simulink model "estimate_gamma_fitting_param"  (R2022a)
settings: Solver=VariableStepAuto  StartTime=0.0  StopTime=tmax  RelTol=1e-3
values from neighbouring files (symbols this model uses):
  c2 = 5    [modelling_parameters.m]
  c2c = c2    (= 5)    [modelling_parameters.m]
  Cr = 2.5    [modelling_parameters.m]
  Eo = 8.41    [modelling_parameters.m]
  K1 = (Voc_min_mes-Eo+K2/soc_min)/-log(100-soc_min)    [modelling_parameters.m]
  K2 = (Voc_max_mes-Eo)*-soc_max    (= 0.99)    [modelling_parameters.m]
  K3 = 1*(-R0+R_soc_min)*soc_min    (= 0.416)    [modelling_parameters.m]
  K3c = 0.02*(-Rc+R_soc_minc)*soc_min    (= 0.00513333333333)    [modelling_parameters.m]
  K4 = 1*(-R0+R_soc_max)*(100-soc_max)    (= -1.45716771982e-16)    [modelling_parameters.m]
  K4c = 2*(-Rc+R_soc_maxc)*(100-soc_max)    (= 0.0733333333333)    [modelling_parameters.m]
  R0 = 0.04    [modelling_parameters.m]
  Rc = 0.03    [modelling_parameters.m]
  Ts = 0.2    [modelling_parameters.m]
settings Model: Creator=spinolam  LastModifiedBy=spinolam

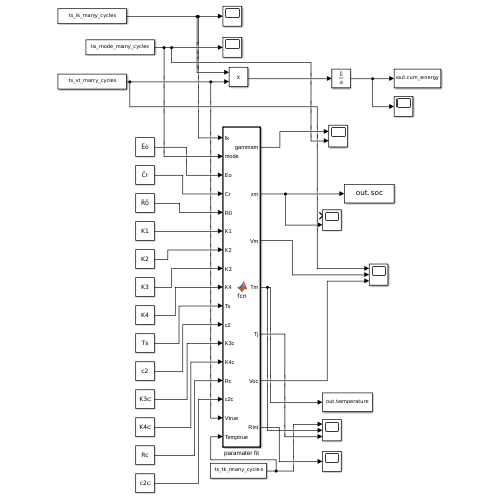
[thumbnail: Simulink's stored preview of the top-level diagram]
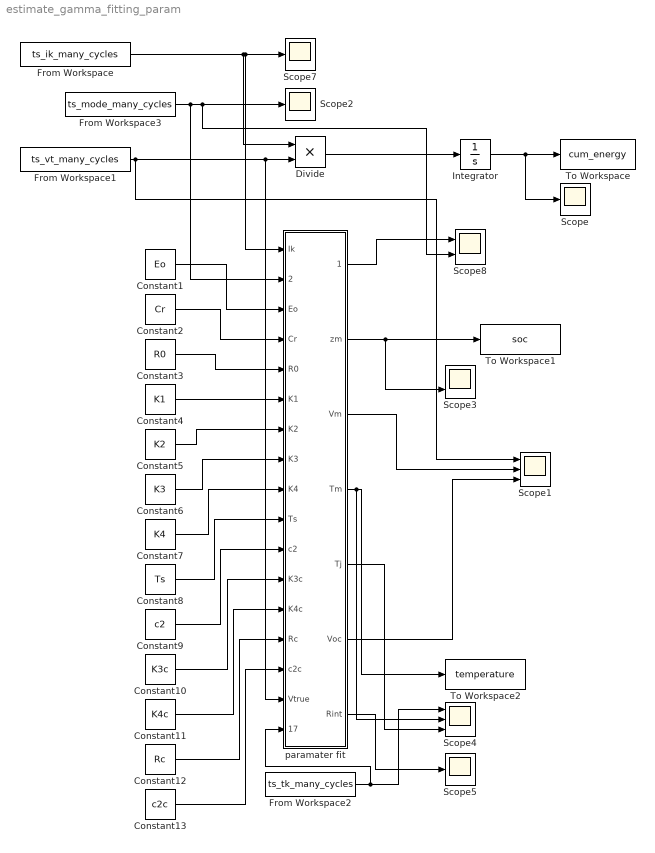
== system estimate_gamma_fitting_param ==
  Constant1 : Constant  Value=Eo
  Constant10 : Constant  Value=K3c
  Constant11 : Constant  Value=K4c
  Constant12 : Constant  Value=Rc
  Constant13 : Constant  Value=c2c
  Constant2 : Constant  Value=Cr
  Constant3 : Constant  Value=R0
  Constant4 : Constant  Value=K1
  Constant5 : Constant  Value=K2
  Constant6 : Constant  Value=K3
  Constant7 : Constant  Value=K4
  Constant8 : Constant  Value=Ts
  Constant9 : Constant  Value=c2
  Divide : Product  Inputs=**
  From Workspace : FromWorkspace  VariableName=ts_ik_many_cycles  SampleTime=Ts
  From Workspace1 : FromWorkspace  VariableName=ts_vt_many_cycles  SampleTime=Ts
  From Workspace2 : FromWorkspace  VariableName=ts_tk_many_cycles  SampleTime=1
  From Workspace3 : FromWorkspace  VariableName=ts_mode_many_cycles  SampleTime=Ts
  Integrator : Integrator
  Scope{,2,5,7} (4 alike) : Scope
  Scope1 : Scope  NumInputPorts=3
  Scope3 : Scope  NumInputPorts=2
  Scope4 : Scope  NumInputPorts=3
  Scope8 : Scope  NumInputPorts=2
  To Workspace : ToWorkspace  VariableName=cum_energy  SampleTime=Ts
  To Workspace1 : ToWorkspace  VariableName=soc  SampleTime=Ts
  To Workspace2 : ToWorkspace  VariableName=temperature  SampleTime=Ts
  paramater fit : MATLAB Function  TreatAsAtomicUnit=on
  wires:
  paramater fit/2(zm) -> To Workspace1/1, Scope3/2
  Integrator/1 -> To Workspace/1, Scope/1
  paramater fit/4(Tm) -> To Workspace2/1, Scope4/2
  Constant13/1 -> paramater fit/15(c2c)
  Constant2/1 -> paramater fit/4(Cr)
  Constant3/1 -> paramater fit/5(R0)
  paramater fit/1(gammam) -> Scope8/1
  paramater fit/7(Rint) -> Scope5/1
  Divide/1 -> Integrator/1
  From Workspace/1 -> Scope7/1, paramater fit/1(Ik), Divide/1
  Constant10/1 -> paramater fit/12(K3c)
  From Workspace3/1 -> Scope8/2, Scope2/1, paramater fit/2(mode)
  Constant11/1 -> paramater fit/13(K4c)
  Constant6/1 -> paramater fit/8(K3)
  paramater fit/6(Voc) -> Scope1/3
  Constant4/1 -> paramater fit/6(K1)
  Constant9/1 -> paramater fit/11(c2)
  Constant8/1 -> paramater fit/10(Ts)
  From Workspace1/1 -> Divide/2, paramater fit/16(Vtrue), Scope1/1
  paramater fit/3(Vm) -> Scope1/2
  Constant1/1 -> paramater fit/3(Eo)
  From Workspace2/1 -> paramater fit/17(Temptrue), Scope4/1
  Constant7/1 -> paramater fit/9(K4)
  Constant5/1 -> paramater fit/7(K2)
  paramater fit/5(Tj) -> Scope4/3
  Constant12/1 -> paramater fit/14(Rc)

== matlab function estimate_gamma_fitting_param/paramater fit ==
  data: Ik input; mode input; gammam output; zm output; Vm output; Tm output; Eo input; Cr input; R0 input; K1 input; K2 input; K3 input; K4 input; Ts input; c2 input; K3c input; K4c input; Rc input; c2c input; Vtrue input; Tj output; Voc output; Rint output; Temptrue input
function [gammam,zm,Vm, Tm,Tj, Voc,Rint]= fcn(Ik,mode,Eo,Cr,R0,K1,K2,K3,K4,Ts,c2,K3c,K4c,Rc,c2c,Vtrue,Temptrue)



persistent zk Vk Tk gammak



z0=99.9;
Tamb=23;
Tj=23;
filtro_gamma=0.999;
Cr=2.6;


%L=1*[-0.6160    0.1816    0.6066];
%L=[-0.0598    0.3907    0.7142];
%L=[-0.0732    0.8348    0.6290];
%L=[-1.3438    5.4291    1.8409];
%L=[-0.5419    3.0073    1.2901];
%L=[-0.0281    2.0100    0.6462];
%L=[-0.3918    6.3832    0.7380];
%L=[-0.2775    6.4987    0.8042];
L=[-0.4207    6.0045    0.7620];
if isempty(gammak)
    gammak=1;
end

if isempty(zk)
    zk=z0;
end

if isempty(Vk) 
    Vk=Eo; 
end

if isempty(Tk)
    Tk=Temptrue; 
    
end

if zk>z0
    zk=z0;
end


if mode==0
    zk=z0;
  %  Vk=Eo;
  %Tk=Temptrue;
    
end


if mode==-1
    error=Vtrue-Vk;

    gamma1=filtro_gamma*gammak + L(1)*error + (1-filtro_gamma)*1;
    
    z1 = zk - Ts*Ik*100*gammak/(3600*Cr)+ L(2)*error;
    
    Rint=(R0+K3/zk+0*K4/(100-zk));
    Voc=Eo-K1*log(100-zk)-K2/zk;
   
    Ek = Voc-(Rint)*Ik*gammak;
    a=exp(-Ts/50);
    V1 = a*Vk + (1-a)*Ek + L(3)*error;

    b=exp(-Ts/ 600);
    Tj= Rint*gammak*Ik^2;
    T1 = b*Tk + (1-b)*(c2*Tj+Tamb);
    
        %sensor model:
    zm = zk; % + noise
    Vm = Vk; % + noise
    gammam =gammak;
    Tm=Tk;
    
    
    %updating z:
    
    zk = z1;
    Vk = V1;
    Tk=T1;
    gammak=gamma1;

elseif mode==1
    error=Vtrue-Vk;

    gamma1=filtro_gamma*gammak + L(1)*error+ (1-filtro_gamma)*1;
    
    z1 = zk - Ts*Ik*100*gammak/(3600*Cr) + L(2)*error;
    
    Rint=(Rc+K3c/zk+K4c/(100-zk)+zk/700);
    Voc=Eo-K1*log(100-zk)-K2/zk;
    V_elec= Rint*Ik;
    Ek = Voc-(Rint)*Ik*gammak;
    a=exp(-Ts/50);
    V1 = a*Vk + (1-a)*Ek + L(3)*error;

    b=exp(-Ts/ 600);
    Tj= Rint*gammak*Ik^2;
    T1 = b*Tk + (1-b)*(c2*Tj+Tamb);
    
        %sensor model:
    zm = zk; % + noise
    Vm = Vk; % + noise
    gammam =gammak;
    Tm=Tk;
    
    
    %updating z:
    
    zk = z1;
    Vk = V1;
    Tk=T1;
    gammak=gamma1;
else
     error=Vtrue-Vk;
%    
%     gamma1=filtro_gamma*gammak + L(1)*error + (1-filtro_gamma)*1;
%     
%     z1 = zk- Ts*Ik*100*gammak/(3600*Cr) + L(2)*error;
%     
     Rint=(R0+K3/zk+K4/(100-zk));
%     
     Voc=Eo-K1*log(100-zk)-K2;
% 
     Ek = Voc-(Rint)*Ik*gammak;
     a=exp(-Ts/50);
     V1 = a*Vk + (1-a)*Ek;
%     
     b=exp(-Ts/600);
     Tj= Rint*gammak*Ik^2;
     T1 = b*Tk + (1-b)*(c2*Tj+Tamb);
% 
%     
%     
%     %updating z:
%     
%     zk = z1;
     Vk = V1;
     Tk=T1;
%     gammak=gamma1;
% 

            %sensor model:
    zm = zk; % + noise
    Vm = Vk; % + noise
    gammam =gammak;
    Tm=Tk;
    
    

end
